simulink model "twelvepulse"  (Simulink 7.5)
settings: Solver=ode45  StartTime=0.0  StopTime=5  RelTol=1e-3
undefined symbols (not defined in the file): D1, Delta, lagging
libraries: powerlib x14, powerlib_extras x1
settings Model: Creator=lm  LastModifiedBy=lm

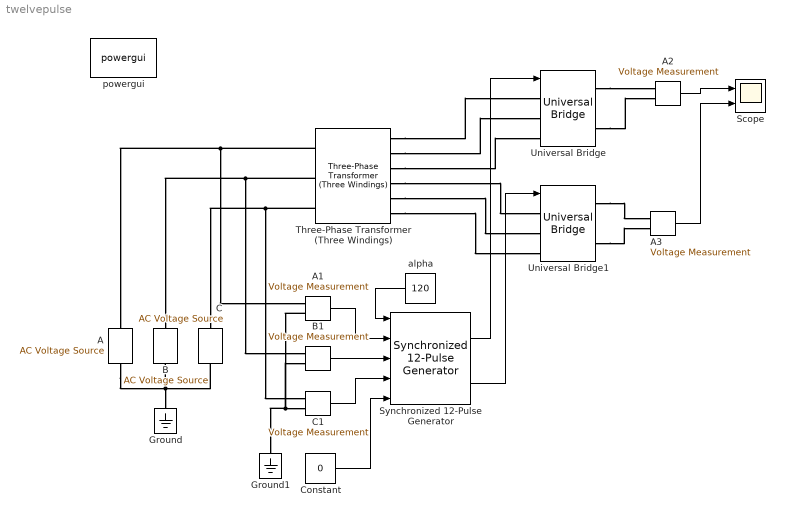
== system twelvepulse ==
  " Synchronized 12-Pulse Generator" : powerlib_extras/Control  Blocks/ Synchronized 12-Pulse Generator  DialogController=POWERSYS.PowerSysDialog  SystemSampleTime=-1  Delta=D1 (lagging)  freq=60  pwidth=20  Double_Pulse=off
  A : powerlib/Electrical Sources/AC Voltage Source  DialogController=POWERSYS.PowerSysDialog  SystemSampleTime=-1  Amplitude=100  Phase=0  Frequency=50  SampleTime=0  Measurements=None
  A1 : powerlib/Measurements/Voltage Measurement  DialogController=POWERSYS.PowerSysDialog  SystemSampleTime=-1  PhasorSimulation=off  OutputType=Complex  PSBequivalent=0
  A2 : powerlib/Measurements/Voltage Measurement  DialogController=POWERSYS.PowerSysDialog  SystemSampleTime=-1  PhasorSimulation=off  OutputType=Complex  PSBequivalent=0
  A3 : powerlib/Measurements/Voltage Measurement  DialogController=POWERSYS.PowerSysDialog  SystemSampleTime=-1  PhasorSimulation=off  OutputType=Complex  PSBequivalent=0
  B : powerlib/Electrical Sources/AC Voltage Source  DialogController=POWERSYS.PowerSysDialog  SystemSampleTime=-1  Amplitude=100  Phase=120  Frequency=50  SampleTime=0  Measurements=None
  B1 : powerlib/Measurements/Voltage Measurement  DialogController=POWERSYS.PowerSysDialog  SystemSampleTime=-1  PhasorSimulation=off  OutputType=Complex  PSBequivalent=0
  C : powerlib/Electrical Sources/AC Voltage Source  DialogController=POWERSYS.PowerSysDialog  SystemSampleTime=-1  Amplitude=100  Phase=240  Frequency=50  SampleTime=0  Measurements=None
  C1 : powerlib/Measurements/Voltage Measurement  DialogController=POWERSYS.PowerSysDialog  SystemSampleTime=-1  PhasorSimulation=off  OutputType=Complex  PSBequivalent=0
  Constant : Constant  Value=0  OutDataType=fixdt(1, 16)  OutScaling=2^0
  Ground : powerlib/Elements/Ground  DialogController=POWERSYS.PowerSysDialog  PhysicalDomain=powersysdomain  SubClassName=unknown  LeftPortType=p1  RightPortType=p1  LConnTagsString=a
  Ground1 : powerlib/Elements/Ground  DialogController=POWERSYS.PowerSysDialog  PhysicalDomain=powersysdomain  SubClassName=unknown  LeftPortType=p1  RightPortType=p1  LConnTagsString=a
  Scope : Scope  NumInputPorts=2
      settings: YMin=0~0  YMax=80~75
  Three-Phase Transformer (Three Windings) : powerlib/Elements/Three-Phase Transformer (Three Windings)  DialogController=POWERSYS.PowerSysDialog  SystemSampleTime=-1  Winding1Connection=Y  UNITS=SI  NominalPower=[ 250e6 , 60 ]  Winding1=[7.35e+005 4.3218 0.45856]  Winding2Connection=Y  Winding2=[3.15e+005 0.7938 0.084225]  Winding3Connection=Delta (D1)  Winding3=[3.15e+005 2.3814 0.25267]  SetSaturation=off  Rm=1.0805e+006  Lm=2866  Saturation=[0 0;0.66653 1910.3;277.72 2419.7]  Hysteresis=off  DataFile='hysteresis'  SetInitialFlux=off  InitialFluxes=[1273.5 -1273.5 1114.3]  Measurements=None  MoreParameters=off  BreakLoop=off  DataType=on  TransfoNumber=1
  Universal Bridge : powerlib/Power Electronics/Universal Bridge  DialogController=POWERSYS.PowerSysDialog  SystemSampleTime=-1  Arms=3  SnubberResistance=1e5  SnubberCapacitance=inf  Device=Thyristors  Ron=1e-3  Lon=0  ForwardVoltages="[  0  0  ]"  ForwardVoltage=0  GTOparameters=[ 10e-6 , 20e-6 ]  IGBTparameters=[ 1e-6 , 2e-6 ]  Measurements=None  Measurements_2=None  converterType=Rectifier
  Universal Bridge1 : powerlib/Power Electronics/Universal Bridge  DialogController=POWERSYS.PowerSysDialog  SystemSampleTime=-1  Arms=3  SnubberResistance=1e5  SnubberCapacitance=inf  Device=Thyristors  Ron=1e-3  Lon=0  ForwardVoltages="[  0  0  ]"  ForwardVoltage=0  GTOparameters=[ 10e-6 , 20e-6 ]  IGBTparameters=[ 1e-6 , 2e-6 ]  Measurements=None  Measurements_2=None  converterType=Rectifier
  alpha : Constant  Value=120  OutDataType=fixdt(1, 16)  OutScaling=2^0
  powergui : powerlib/powergui  Priority=1  SystemSampleTime=-1  SimulationMode=Discrete  SampleTime=50e-6  frequency=60  SPID=off  DisableSnubberDevices=off  DisableRonSwitches=off  DisableVfSwitches=off  SwTol=0  Interpol=off  frequencyindice=50  echomessages=off  HookPort=off  DisplayEquations=off  FunctionMessages=off  EnableUseOfTLC=off  x0status=blocks  RestoreLinks=warning  ResistiveCurrentMeasurement=off  Ylog=off  Xlog=on  ShowGrid=off  save=off  variable=ZData  ZoomFFT=off  StartTime=0.0  cycles=1  DisplayStyle=1  FreqAxis=off  MaxFrequency=1000  frequencyindicesteady=1  display=off  methode=off
  wires:
  A1/1 -> " Synchronized 12-Pulse Generator"/2
  B1/1 -> " Synchronized 12-Pulse Generator"/3
  C1/1 -> " Synchronized 12-Pulse Generator"/4
  " Synchronized 12-Pulse Generator"/1 -> Universal Bridge/1
  " Synchronized 12-Pulse Generator"/2 -> Universal Bridge1/1
  Constant/1 -> " Synchronized 12-Pulse Generator"/5
  alpha/1 -> " Synchronized 12-Pulse Generator"/1
  A2/1 -> Scope/1
  A3/1 -> Scope/2
  connections:
  A/LConn1 -- B/LConn1 -- C/LConn1 -- Ground/LConn1
  Three-Phase Transformer (Three Windings)/LConn3 -- C/RConn1 -- C1/LConn1
  Three-Phase Transformer (Three Windings)/LConn2 -- B/RConn1 -- B1/LConn1
  Three-Phase Transformer (Three Windings)/LConn1 -- A/RConn1 -- A1/LConn1
  Three-Phase Transformer (Three Windings)/RConn1 -- Universal Bridge/LConn1
  Three-Phase Transformer (Three Windings)/RConn2 -- Universal Bridge/LConn2
  Three-Phase Transformer (Three Windings)/RConn3 -- Universal Bridge/LConn3
  Three-Phase Transformer (Three Windings)/RConn4 -- Universal Bridge1/LConn1
  Three-Phase Transformer (Three Windings)/RConn5 -- Universal Bridge1/LConn2
  Three-Phase Transformer (Three Windings)/RConn6 -- Universal Bridge1/LConn3
  A1/LConn2 -- B1/LConn2 -- C1/LConn2 -- Ground1/LConn1
  Universal Bridge/RConn1 -- A2/LConn1
  Universal Bridge/RConn2 -- A2/LConn2
  Universal Bridge1/RConn2 -- A3/LConn2
  Universal Bridge1/RConn1 -- A3/LConn1
